simulink model "k1visey"  (Simulink 8.5)
settings: Solver=ode45  StartTime=0.0  StopTime=10.0  RelTol=1e-3
libraries: cdsFilt x6, cdsIPCx x5, cdsEpicsOut x3, cdsAdcx0 x1, dac x1, TYPEC_MASTER x1, cdsParameters x1
settings Model: Creator=controls  LastModifiedBy=controls
settings DataIOCC: SignalLoggingSaveFormat=Dataset
settings OptimizationCC: ExpressionDepthLimit=128
settings DebuggingCC: UnderspecifiedInitializationDetection=Simplified  MergeDetectMultiDrivingBlocksExec=error  FcnCallInpInsideContextMsg=EnableAllAsError  StateNameClashWarn=none
settings GRTTargetCC: CombineOutputUpdateFcns=on  GRTInterface=off

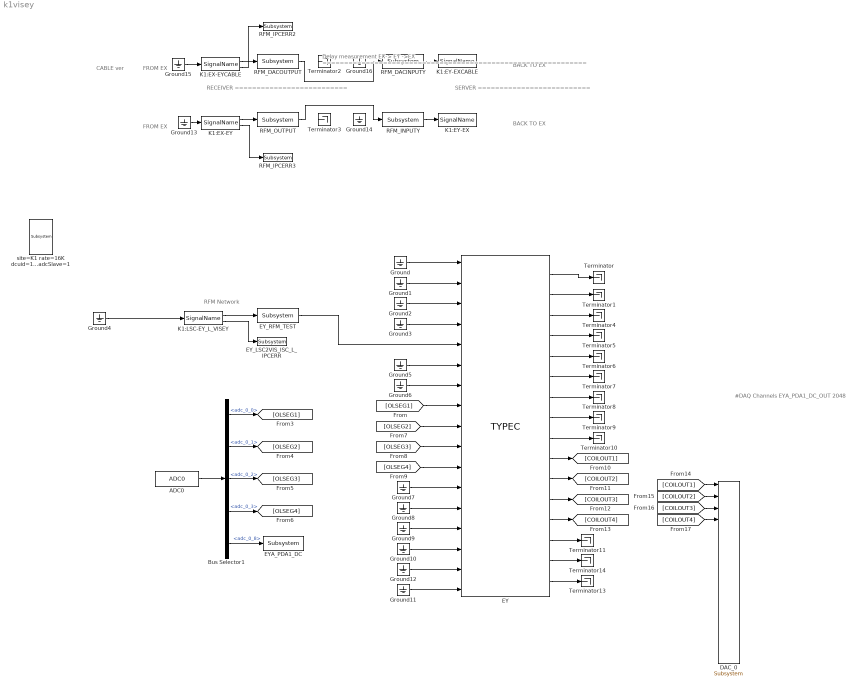
== system k1visey ==
  note: RFM Network
  note: #DAQ Channels
      |
      | EYA_PDA1_DC_OUT 2048
  note: FROM EX
  note: CABLE ver
  note: BACK TO EX
  note: FROM EX
  note: BACK TO EX
  note: Delay measurement
      | EX-> EY ->EX
      | =============================================================
  note: SERVER
      | ==========================
  note: RECEIVER
      | ==========================
  ADC0 : cdsAdcx0/ADC0  Tag=cdsAdc  Description=|
      | type-GSC_16AI64SSA
      | card_num=0
      settings: AttributesFormatString=%<Description>\n%<Tag>
  Bus Selector1 : BusSelector  Description=ADC Selector  OutputSignals=adc_0_0,adc_0_1,adc_0_2,adc_0_3,adc_0_8
      settings: AttributesFormatString=%<Description>
  DAC_0 : dac/Subsystem  Description=|
      | type=GSC_16AO16,
      | card_num=0
      settings: AttributesFormatString=%<Description>
  EY : TYPEC_MASTER/TYPEC  Description=TYPEC MASTER
      settings: AttributesFormatString=%<Description>
  EYA_PDA1_DC : cdsFilt/Subsystem  Tag=cdsFilt  Description=|
      | Purpose:                                                                                                                                                                                                                                  
      | Standard CDS IIR filter module.                                                                                                                                                                                                           
      |                                                                                                                                                                                                                                           
      | Operation:                                                                                                                                                                                                                                
      | Consists of 10 second order section IIR filters, plus a ramped gain stage. In FE code, also provides pre-defined test points and excitation channel inputs. The filter coefficients are defined in the LIGO system using the 'foton' tool.
      |                                                                                                                                                                                                                                           
      | Usage:                                                                                                                                                                                                                                    
      | Name the part with the desired filter module name.
      settings: AttributesFormatString=%<Tag>
  EY_LSC2VIS_ISC_L_IPCERR : cdsEpicsOut/Subsystem  Tag=cdsEpicsOutput  Description=|
      | Purpose:                                          
      | Output a FE signal to an EPICS channel.           
      |                                                   
      | Operation:                                        
      | Takes input value and passes it to EPICS record.  
      |                                                   
      | Usage:                                            
      | Name the part with the desired EPICS rrecord name.
      settings: AttributesFormatString=%<Tag>
  EY_RFM_TEST : cdsFilt/Subsystem  Tag=cdsFilt  Description=|
      | Purpose:                                                                                                                                                                                                                                  
      | Standard CDS IIR filter module.                                                                                                                                                                                                           
      |                                                                                                                                                                                                                                           
      | Operation:                                                                                                                                                                                                                                
      | Consists of 10 second order section IIR filters, plus a ramped gain stage. In FE code, also provides pre-defined test points and excitation channel inputs. The filter coefficients are defined in the LIGO system using the 'foton' tool.
      |                                                                                                                                                                                                                                           
      | Usage:                                                                                                                                                                                                                                    
      | Name the part with the desired filter module name.
      settings: AttributesFormatString=%<Tag>
  Ground{,1..16} (17 alike) : Ground
  K1:EX-EY : cdsIPCx/SignalName  Tag=cdsIPCx_RFM  Description=card=0
      settings: AttributesFormatString=%<Description>\n%<Tag>
  K1:EX-EYCABLE : cdsIPCx/SignalName  Tag=cdsIPCx_RFM  Description=card=0
      settings: AttributesFormatString=%<Description>\n%<Tag>
  K1:EY-EX : cdsIPCx/SignalName  Tag=cdsIPCx_RFM  Description=card=0
      settings: AttributesFormatString=%<Description>\n%<Tag>
  K1:EY-EXCABLE : cdsIPCx/SignalName  Tag=cdsIPCx_RFM  Description=card=0
      settings: AttributesFormatString=%<Description>\n%<Tag>
  K1:LSC-EY_L_VISEY : cdsIPCx/SignalName  Tag=cdsIPCx_RFM  Description=card=0
      settings: AttributesFormatString=%<Description>\n%<Tag>
  RFM_DACINPUTY : cdsFilt/Subsystem  Tag=cdsFilt  Description=|
      | Purpose:                                                                                                                                                                                                                                  
      | Standard CDS IIR filter module.                                                                                                                                                                                                           
      |                                                                                                                                                                                                                                           
      | Operation:                                                                                                                                                                                                                                
      | Consists of 10 second order section IIR filters, plus a ramped gain stage. In FE code, also provides pre-defined test points and excitation channel inputs. The filter coefficients are defined in the LIGO system using the 'foton' tool.
      |                                                                                                                                                                                                                                           
      | Usage:                                                                                                                                                                                                                                    
      | Name the part with the desired filter module name.
      settings: AttributesFormatString=%<Tag>
  RFM_DACOUTPUT : cdsFilt/Subsystem  Tag=cdsFilt  Description=|
      | Purpose:                                                                                                                                                                                                                                  
      | Standard CDS IIR filter module.                                                                                                                                                                                                           
      |                                                                                                                                                                                                                                           
      | Operation:                                                                                                                                                                                                                                
      | Consists of 10 second order section IIR filters, plus a ramped gain stage. In FE code, also provides pre-defined test points and excitation channel inputs. The filter coefficients are defined in the LIGO system using the 'foton' tool.
      |                                                                                                                                                                                                                                           
      | Usage:                                                                                                                                                                                                                                    
      | Name the part with the desired filter module name.
      settings: AttributesFormatString=%<Tag>
  RFM_INPUTY : cdsFilt/Subsystem  Tag=cdsFilt  Description=|
      | Purpose:                                                                                                                                                                                                                                  
      | Standard CDS IIR filter module.                                                                                                                                                                                                           
      |                                                                                                                                                                                                                                           
      | Operation:                                                                                                                                                                                                                                
      | Consists of 10 second order section IIR filters, plus a ramped gain stage. In FE code, also provides pre-defined test points and excitation channel inputs. The filter coefficients are defined in the LIGO system using the 'foton' tool.
      |                                                                                                                                                                                                                                           
      | Usage:                                                                                                                                                                                                                                    
      | Name the part with the desired filter module name.
      settings: AttributesFormatString=%<Tag>
  RFM_IPCERR2 : cdsEpicsOut/Subsystem  Tag=cdsEpicsOutput  Description=|
      | Purpose:                                          
      | Output a FE signal to an EPICS channel.           
      |                                                   
      | Operation:                                        
      | Takes input value and passes it to EPICS record.  
      |                                                   
      | Usage:                                            
      | Name the part with the desired EPICS rrecord name.
      settings: AttributesFormatString=%<Tag>
  RFM_IPCERR3 : cdsEpicsOut/Subsystem  Tag=cdsEpicsOutput  Description=|
      | Purpose:                                          
      | Output a FE signal to an EPICS channel.           
      |                                                   
      | Operation:                                        
      | Takes input value and passes it to EPICS record.  
      |                                                   
      | Usage:                                            
      | Name the part with the desired EPICS rrecord name.
      settings: AttributesFormatString=%<Tag>
  RFM_OUTPUT : cdsFilt/Subsystem  Tag=cdsFilt  Description=|
      | Purpose:                                                                                                                                                                                                                                  
      | Standard CDS IIR filter module.                                                                                                                                                                                                           
      |                                                                                                                                                                                                                                           
      | Operation:                                                                                                                                                                                                                                
      | Consists of 10 second order section IIR filters, plus a ramped gain stage. In FE code, also provides pre-defined test points and excitation channel inputs. The filter coefficients are defined in the LIGO system using the 'foton' tool.
      |                                                                                                                                                                                                                                           
      | Usage:                                                                                                                                                                                                                                    
      | Name the part with the desired filter module name.
      settings: AttributesFormatString=%<Tag>
  Terminator{,1..11,13..14} (14 alike) : Terminator
  site=K1 rate=16K dcuid=106 host=k1ey0 specific_cpu=3 adcSlave=1 : cdsParameters/Subsystem  Tag=cdsParameters  Description=|
      | Purpose:                                                                                                                                                                                                                                
      | Provide system parameters to the FE code generator to properly configure the generated EPICS names, rep rate of the FE controller, and the Data Acquisition node ID for proper storage of data from this FE controller.                 
      |                                                                                                                                                                                                                                         
      | Useage:                                                                                                                                                                                                                                 
      | The part NAME field is used to identify the FE parameters. It must be of the form:                                                                                                                                                      
      | site=                                                                                                                                                                                                                                   
      | rate=                                                                                                                                                                                                                                   
      | dcuid=                                                                                                                                                                                                                                  
      |                                                                                                                                                                                                                                         
      | Where:                                                                                                                                                                                                                                  
      | site= argument may be H1, H2, L1, M1, G1, either as a single argument or multiple, for example site=H1,H2. These are the only names allowed. These will become the first two characters of all EPICS and signal names (for example G1:).
      |                                                                                                                                                                                                                                         
      | rate= may be 2K, 16K, 32K, or 64K                                                                                                                                                                                                       
      |                                                                                                                                                                                                                                         
      | dcuid= is site specific ie it must be unique at each site.
      settings: AttributesFormatString=%<Tag>
  wires:
  Ground2/1 -> EY/3
  Ground1/1 -> EY/2
  Ground/1 -> EY/1
  Ground3/1 -> EY/4
  Ground8/1 -> EY/13
  Ground7/1 -> EY/12
  Ground9/1 -> EY/14
  Ground10/1 -> EY/15
  K1:LSC-EY_L_VISEY/1 -> EY_RFM_TEST/1
  Ground5/1 -> EY/6
  Ground12/1 -> EY/16
  Ground11/1 -> EY/17
  EY/1 -> Terminator/1
  EY/2 -> Terminator1/1
  EY/5 -> Terminator6/1
  EY/4 -> Terminator5/1
  EY/6 -> Terminator7/1
  EY/3 -> Terminator4/1
  EY/7 -> Terminator8/1
  EY/9 -> Terminator10/1
  EY/8 -> Terminator9/1
  EY/14 -> Terminator11/1
  EY/15 -> Terminator14/1
  EY/16 -> Terminator13/1
  Ground6/1 -> EY/7
  K1:LSC-EY_L_VISEY/2 -> EY_LSC2VIS_ISC_L_IPCERR/1
  ADC0/1 -> Bus Selector1/1
  Bus Selector1/5 -> EYA_PDA1_DC/1  "<adc_0_8>"
  Ground4/1 -> K1:LSC-EY_L_VISEY/1
  EY_RFM_TEST/1 -> EY/5
  Bus Selector1/3 -> [OLSEG3]  "<adc_0_2>"
  Bus Selector1/1 -> [OLSEG1]  "<adc_0_0>"
  Bus Selector1/4 -> [OLSEG4]  "<adc_0_3>"
  Bus Selector1/2 -> [OLSEG2]  "<adc_0_1>"
  [OLSEG1] -> EY/8
  [OLSEG2] -> EY/9
  [OLSEG4] -> EY/11
  [OLSEG3] -> EY/10
  [COILOUT1] -> DAC_0/1
  [COILOUT2] -> DAC_0/2
  [COILOUT3] -> DAC_0/3
  [COILOUT4] -> DAC_0/4
  EY/10 -> [COILOUT1]
  EY/11 -> [COILOUT2]
  EY/12 -> [COILOUT3]
  EY/13 -> [COILOUT4]
  K1:EX-EY/1 -> RFM_OUTPUT/1
  K1:EX-EY/2 -> RFM_IPCERR3/1
  Ground13/1 -> K1:EX-EY/1
  RFM_INPUTY/1 -> K1:EY-EX/1
  RFM_OUTPUT/1 -> RFM_INPUTY/1
  K1:EX-EYCABLE/1 -> RFM_DACOUTPUT/1
  K1:EX-EYCABLE/2 -> RFM_IPCERR2/1
  Ground15/1 -> K1:EX-EYCABLE/1
  RFM_DACINPUTY/1 -> K1:EY-EXCABLE/1
  RFM_DACOUTPUT/1 -> RFM_DACINPUTY/1
